simulink model "lab3_step2"  (R2019b)
settings: Solver=VariableStepAuto  StartTime=0.0  StopTime=5  RelTol=1e-3
InitFcn:
  | W_bits = 32;
  | F_bits = 16;
  | 
  | p = 1;
  | q = 1;
  | 
  | filename ='C:\Users\Louis\Desktop\SoC-FPGAs-II\Lab 3\green_day.wav';
  | 
  | [y,Fs] = audioread(filename);
  | 
  | input_signal = resample(y,p,q);
  | 
  | t = zeros(length(input_signal),1);
  | 
  | for i = 1:length(input_signal)
  |  t(i) = 1/Fs * i*q;
  | end
  | 
  | input_signal = [t input_signal];
StopFcn:
  | output_signal = [out.tout out.output_signal];
  | 
  | sound(output_signal,Fs);
undefined symbols (not defined in the file): Fs, magnitude
libraries: dspstat3 x2
settings Model: Creator=Louis  LastModifiedBy=Louis

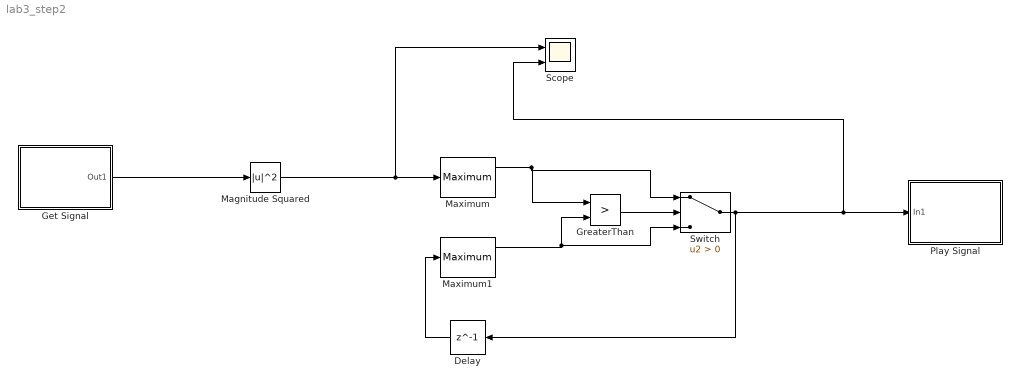
== system lab3_step2 ==
  Delay : Delay  DelayLength=1
  Get Signal : Subsystem
  GreaterThan : RelationalOperator  Operator=>  OutDataTypeStr=boolean  RndMeth=Simplest
  Magnitude Squared : Math  Operator=magnitude^2  SignedPower=off  SaturateOnIntegerOverflow=on
  Maximum : dspstat3/Maximum  operation=maximum  fcn=Value and Index  indexBase=One  operateOver=Each column  Dimension=1  InputProcessing=Columns as channels (frame based)  reset=None  roiEnable=off  roiType=Rectangles  roiPortion=Entire ROI  roiOutput=Individual statistics for each ROI  roiFlag=off  roundingMode=Floor  overflowMode=off  accumDataTypeStr=Inherit: Same as product output  accumLastDataTypeStr=Inherit: Same as product output
  Maximum1 : dspstat3/Maximum  operation=maximum  fcn=Value and Index  indexBase=One  operateOver=Each column  Dimension=1  InputProcessing=Columns as channels (frame based)  reset=None  roiEnable=off  roiType=Rectangles  roiPortion=Entire ROI  roiOutput=Individual statistics for each ROI  roiFlag=off  roundingMode=Floor  overflowMode=off  accumDataTypeStr=Inherit: Same as product output  accumLastDataTypeStr=Inherit: Same as product output
  Play Signal : Subsystem
  Scope : Scope  NumInputPorts=2
  Switch : Switch  Criteria=u2 > Threshold
  wires:
  Get Signal/1(Out1) -> Magnitude Squared/1
  Magnitude Squared/1 -> Maximum/1, Scope/1
  Maximum/1 -> Switch/1, GreaterThan/1
  Delay/1 -> Maximum1/1
  Maximum1/1 -> Switch/3, GreaterThan/2
  GreaterThan/1 -> Switch/2
  Switch/1 -> Delay/1, Scope/2, Play Signal/1(In1)

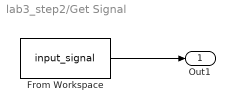
== system lab3_step2/Get Signal ==
  From Workspace : FromWorkspace  VariableName=input_signal  OutDataTypeStr=double  SampleTime=1/Fs*q*4
  Out1 : Outport
  wires:
  From Workspace/1 -> Out1/1

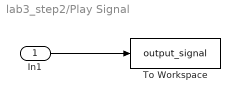
== system lab3_step2/Play Signal ==
  In1 : Inport
  To Workspace : ToWorkspace  VariableName=output_signal  SampleTime=1/Fs
      settings: Save2DSignal=2-D array (concatenate along first dimension)
  wires:
  In1/1 -> To Workspace/1
